simulink model "cndiag"  (Simulink 6.5)
settings: Solver=ode45  SolverMode=SingleTasking  StartTime=0.0  StopTime=999999  MaxStep=10  RelTol=1e-3  AbsTol=1e-3
undefined symbols (not defined in the file): k, TI
settings Model: Creator=lfd  LastModifiedBy=lfd  ExtModeAutoUpdateStatusClock=off
settings DataIOCC: LimitDataPoints=off  SaveOutput=off  SaveTime=off
settings OptimizationCC: BlockReduction=off  BooleanDataType=off
settings DebuggingCC: SolverPrmCheckMsg=none  MultiTaskDSMMsg=warning  MultiTaskCondExecSysMsg=none  StrictBusMsg=None
settings HardwareCC: TargetUnknown=on
settings RTWCC: IncludeERTFirstTime=on
settings GRTTargetCC: ModelReferenceCompliant=off  MatFileLogging=off

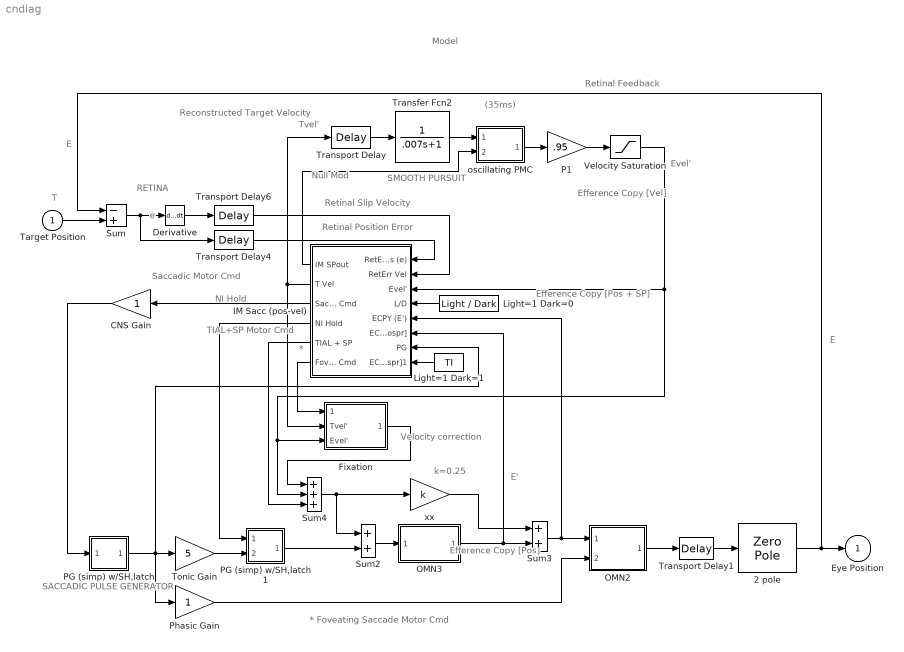
== system cndiag ==
  note: TIAL+SP
      | Motor
      | Cmd
  note: Tvel'
  note: RETINA
  note: Efference Copy
      | [Pos + SP]
  note: Retinal Position Error
  note: SACCADIC
      | PULSE
      | GENERATOR
  note: NI Hold
  note: (35ms)
  note: Model
  note: SMOOTH PURSUIT
  note: Efference Copy
      | [Vel]
  note: Reconstructed
      | Target Velocity
  note: Retinal Feedback
  note: E
  note: Saccadic
      |  Motor Cmd
  note: Evel'
  note: e
  note: Retinal Slip Velocity
  note: E
  note: T
  note: E'
  note: Efference
      | Copy
      | [Pos]
  note: Velocity
      | correction
  note: k=0.25
  note: *
  note: * Foveating Saccade Motor Cmd
  note: Null Mod
  Target Position : Inport
  2 pole : ZeroPole  Zeros=[ ]  Poles=[ -1/.18 -1/.007]  Gain=[1/.18 * 1/.007]
      mask Display: disp('EOM\n[2-Pole\nPlant]')
  CNS Gain : Gain  Orientation=left  SaturateOnIntegerOverflow=on
  Derivative : Derivative
      mask Display: disp('s')
  Fixation : Subsystem
      mask Display: disp('Fixation')
  IM Sacc (pos-vel) : Subsystem  Orientation=left
      mask Display: disp('INTERNAL\nMONITOR\n[Sacc,SP,AL,\nNI Control]')
  Light=1 Dark=0 : Constant  Orientation=left  Value=Light / Dark
  Light=1 Dark=1 : Constant  Orientation=left  Value=TI
  OMN2 : Subsystem
      mask Display: disp('OMN\n[Tonic +\nPhasic]')
  OMN3 : Subsystem
      mask Display: disp('Neural \nIntegrator')
  P1 : Gain  Gain=.95  SaturateOnIntegerOverflow=on
  PG (simp) w/SH,latch : Subsystem
      mask Display: disp('PG')
  PG (simp) w/SH,latch1 : Subsystem
      mask Display: disp('NI\nHold')
  Phasic Gain : Gain  SaturateOnIntegerOverflow=on
  Sum : Sum  Inputs=-+  SaturateOnIntegerOverflow=on  InputSameDT=on
  Sum2 : Sum  SaturateOnIntegerOverflow=on  InputSameDT=on
  Sum3 : Sum  SaturateOnIntegerOverflow=on  InputSameDT=on
  Sum4 : Sum  Inputs=+++  SaturateOnIntegerOverflow=on  InputSameDT=on
  Tonic Gain : Gain  Gain=5  SaturateOnIntegerOverflow=on
  Transfer Fcn2 : TransferFcn  Denominator=[.007 1]
  Transport Delay : TransportDelay  DelayTime=0.015
      mask Display: disp('15ms')
  Transport Delay1 : TransportDelay  DelayTime=0.03
      mask Display: disp('30ms')
  Transport Delay4 : TransportDelay  DelayTime=.05
      mask Display: disp('50ms')
  Transport Delay6 : TransportDelay  DelayTime=.05
      mask Display: disp('50ms')
  Velocity Saturation : Saturate  UpperLimit=90  LowerLimit=-90
  oscillating PMC : Subsystem
      mask Display: disp('PMC+')
  xx : Gain  Gain=k  SaturateOnIntegerOverflow=on
  Eye Position : Outport  InitialOutput=0
  wires:
  Transport Delay4/1 -> IM Sacc (pos-vel)/1(RetErr Pos (e))
  Transport Delay/1 -> Transfer Fcn2/1
  oscillating PMC/1(efference copy eye vel) -> P1/1
  P1/1 -> Velocity Saturation/1
  Transfer Fcn2/1 -> oscillating PMC/1(desired eye vel)
  Target Position/1 -> Sum/2
  Light=1 Dark=0/1 -> IM Sacc (pos-vel)/4(L/D)
  Sum/1 -> Derivative/1, Transport Delay4/1
  Transport Delay6/1 -> IM Sacc (pos-vel)/2(RetErr Vel)
  Derivative/1 -> Transport Delay6/1
  Velocity Saturation/1 -> IM Sacc (pos-vel)/3(Evel'), Sum4/2, Fixation/3(Evel')
  Tonic Gain/1 -> PG (simp) w/SH,latch1/2(in_2)
  PG (simp) w/SH,latch/1(out_1) -> Phasic Gain/1, Tonic Gain/1, IM Sacc (pos-vel)/7(PG)
  OMN3/1(out_1) -> IM Sacc (pos-vel)/6(ECPY [epospr]), Sum3/2
  PG (simp) w/SH,latch1/1(out_1) -> Sum2/2
  Phasic Gain/1 -> OMN2/2(from PG)
  Sum2/1 -> OMN3/1(from NI)
  xx/1 -> Sum3/1
  Sum3/1 -> OMN2/1(from NI), IM Sacc (pos-vel)/5(ECPY (E'))
  2 pole/1 -> Eye Position/1, Sum/1
  Transport Delay1/1 -> 2 pole/1
  OMN2/1(out_1) -> Transport Delay1/1
  Sum4/1 -> xx/1, Sum2/1
  CNS Gain/1 -> PG (simp) w/SH,latch/1(in_1)
  Fixation/1(" CorrVel [velcorr]") -> Sum4/1
  Light=1 Dark=1/1 -> IM Sacc (pos-vel)/8(ECPY [epospr]1)
  IM Sacc (pos-vel)/6(Fov Sac Mot Cmd) -> Fixation/1(fs [fsmc30])
  IM Sacc (pos-vel)/1(IM SPout) -> oscillating PMC/2(Null mod)
  IM Sacc (pos-vel)/2(T Vel) -> Transport Delay/1, Fixation/2(Tvel')
  IM Sacc (pos-vel)/5(TIAL + SP) -> Sum4/3
  IM Sacc (pos-vel)/4(NI Hold) -> PG (simp) w/SH,latch1/1(in_1)
  IM Sacc (pos-vel)/3(Sac Mot Cmd) -> CNS Gain/1

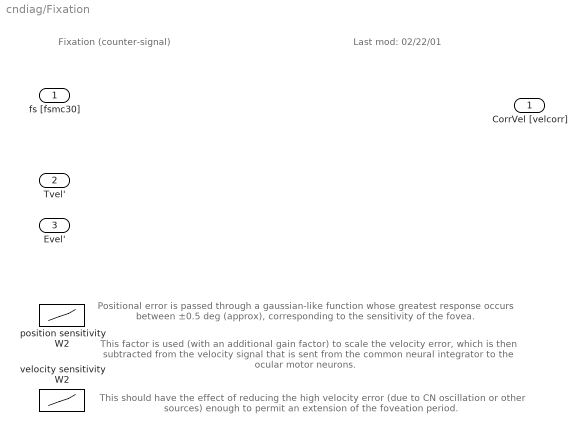
== system cndiag/Fixation ==
  note: Fixation (counter-signal)
  note: Last mod: 02/22/01
  note: Positional error is passed through a gaussian-like function whose greatest
      | response occurs between ±0.5 deg (approx), corresponding to the sensitivity
      | of the fovea.
  note: This factor is used (with an additional gain factor) to scale the velocity error,
      | which is then subtracted from the velocity signal that is sent from the
      | common neural integrator to the ocular motor neurons.
  note: This should have the effect of reducing the high velocity error (due
      | to CN oscillation or other sources) enough to permit an extension of
      | the foveation period.
  fs [fsmc30] : Inport
  Tvel' : Inport  Port=2
  Evel' : Inport  Port=3
  position sensitivity W2 : Lookup  InputValues="[-5 -2  -1 -0.5   0.5   1    2    5]"  OutputValues="[ 0   0.125    0.5     1      1     0.5    0.125  0]"  SaturateOnIntegerOverflow=on
  velocity sensitivity W2 : Lookup  InputValues="[-30 -15   -8  -4   4     8  15  30]"  OutputValues="[0  0.125   0.5    1    1    0.5   0.125  0]"  SaturateOnIntegerOverflow=on
  " CorrVel [velcorr]" : Outport  InitialOutput=0
  wires:
  ? -> " CorrVel [velcorr]"/1

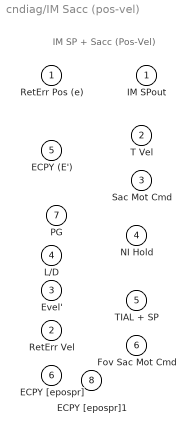
== system cndiag/IM Sacc (pos-vel) ==
  note: IM SP + Sacc (Pos-Vel)
  RetErr Pos (e) : Inport
  RetErr Vel : Inport  Port=2
  Evel' : Inport  Port=3
  L/D : Inport  Port=4
  ECPY (E') : Inport  Port=5
  ECPY [epospr] : Inport  Port=6
  PG : Inport  Port=7
  ECPY [epospr]1 : Inport  Port=8
  IM SPout : Outport  InitialOutput=0
  T Vel : Outport  Port=2  InitialOutput=0
  Sac Mot Cmd : Outport  Port=3  InitialOutput=0
  NI Hold : Outport  Port=4  InitialOutput=0
  TIAL + SP : Outport  Port=5  InitialOutput=0
  Fov Sac Mot Cmd : Outport  Port=6  InitialOutput=0

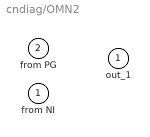
== system cndiag/OMN2 ==
  from NI : Inport
  from PG : Inport  Port=2
  out_1 : Outport  InitialOutput=0

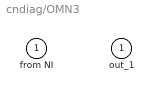
== system cndiag/OMN3 ==
  from NI : Inport
  out_1 : Outport  InitialOutput=0

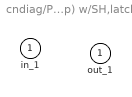
== system cndiag/PG (simp) w/SH,latch ==
  in_1 : Inport
  out_1 : Outport  InitialOutput=0

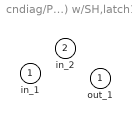
== system cndiag/PG (simp) w/SH,latch1 ==
  in_1 : Inport
  in_2 : Inport  Port=2
  out_1 : Outport  InitialOutput=0

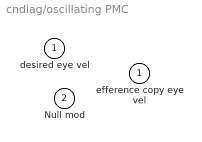
== system cndiag/oscillating PMC ==
  desired eye vel : Inport
  Null mod : Inport  Port=2
  efference copy eye vel : Outport  InitialOutput=0
